simulink model "pcontrol"  (R2019b)
settings: Solver=VariableStepAuto  StartTime=0.0  StopTime=10.0  RelTol=1e-3
values from neighbouring files (symbols this model uses):
  b = 2.61*10^-4    (= 0.000261)    [params.m]
  J_m = 5.62*10^-5    (= 5.62e-05)    [params.m]
  K_e = 0.068    [params.m]
  K_p = k    [params.m]
  K_t = 0.068    [params.m]
  K_Tach = 0.134    [params.m]
  L_a = 3*10^-3    (= 0.003)    [params.m]
  R_a = 1.63    [params.m]
  T_mech = i    [params.m]
  V_sig = 7    [params.m]
settings Model: Creator=Jasper  LastModifiedBy=Jasper

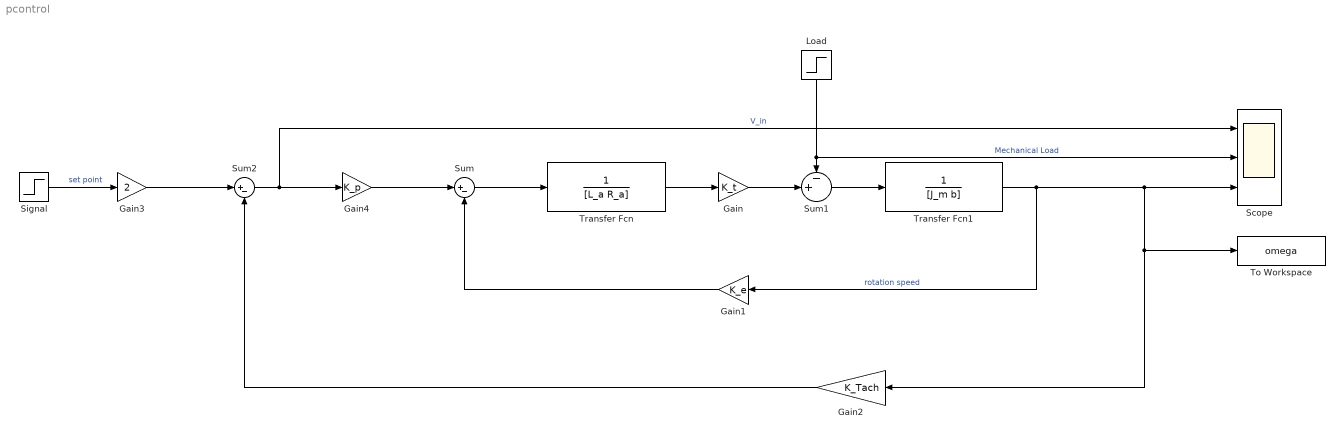
== system pcontrol ==
  Gain : Gain  Gain=K_t
  Gain1 : Gain  Gain=K_e
  Gain2 : Gain  Gain=K_Tach
  Gain3 : Gain  Gain=2
  Gain4 : Gain  Gain=K_p
  Load : Step  Time=3  After=T_mech  SampleTime=0
  Scope : Scope  NumInputPorts=3
  Signal : Step  Time=0  After=V_sig  SampleTime=0
  Sum : Sum  Inputs=|+-
  Sum1 : Sum  Inputs=-+|
  Sum2 : Sum  Inputs=|+-
  To Workspace : ToWorkspace  VariableName=omega  SaveFormat=Timeseries  SampleTime=-1
  Transfer Fcn : TransferFcn  Denominator=[L_a R_a]
  Transfer Fcn1 : TransferFcn  Denominator=[J_m b]
  wires:
  Sum/1 -> Transfer Fcn/1
  Gain1/1 -> Sum/2
  Transfer Fcn1/1 -> Gain1/1, To Workspace/1, Gain2/1, Scope/3  "rotation speed"
  Sum1/1 -> Transfer Fcn1/1
  Gain/1 -> Sum1/2
  Transfer Fcn/1 -> Gain/1
  Load/1 -> Scope/2, Sum1/1  "Mechanical Load"
  Gain2/1 -> Sum2/2
  Sum2/1 -> Gain4/1, Scope/1  "V_in"
  Signal/1 -> Gain3/1  "set point"
  Gain3/1 -> Sum2/1
  Gain4/1 -> Sum/1
